simulink model "doc_fmsampletime"  (Simulink 5.0)
settings: Solver=ode45  StartTime=0.0  StopTime=10.0  RelTol=1e-3
undefined symbols (not defined in the file): slcm
libraries: commanapbnd2 x1
settings Model: CovMetricSettings=d  Creator=agaltman  LastModifiedBy=agaltman  SignalLoggingName=logsOut  BlockReductionOpt=off  BooleanDataType=off  ZeroCrossControl=UseLocalSettings  RTWMathFcnLibMatFile=iso_c_tmw.mat

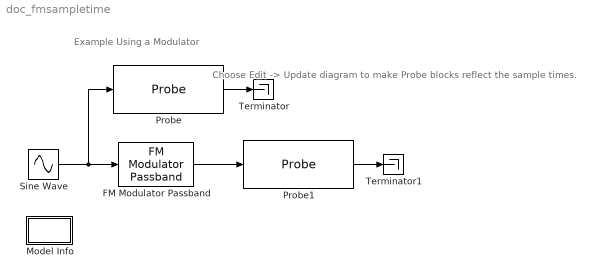
== system doc_fmsampletime ==
  note: Example Using a Modulator
  note: Choose Edit -> Update diagram
      | to make Probe blocks reflect
      | the sample times.
  FM Modulator Passband : commanapbnd2/FM Modulator Passband  Fc=100  Ph=0  HzPerV=1  ts=1  td=Inf
  Model Info : Subsystem  LoadFcn=slcm LoadBlock;  InitFcn=slcm('UpdateAllCMBlocksInThisModelInit')  mask(CMBlock){InitialSaveTempField=, InitialBlockCM=none, BlockCM=none, Frame=on, SaveTempField=, DisplayStringWithTags=Info, MaskDisplayString=Info, HorizontalTextAlignment=Center, LeftAlignmentValue=0.5, SourceBlockDiagram=doc_fmsampletime, TagMaxNumber=20, CMTag1=, CMTag2=, CMTag3=, CMTag4=, CMTag5=, CMTag6=, CMTag7=, CMTag8=, CMTag9=, CMTag10=, CMTag11=, CMTag12=, CMTag13=, CMTag14=, CMTag15=, CMTag16=, CMTag17=, CMTag18=, CMTag19=, CMTag20=}
      mask help: This block allows revision control information to be displayed within the model.
      settings: CopyFcn=slcm CopyBlock;  DeleteFcn=slcm Cancel;  PostSaveFcn=slcm('UpdateAllCMBlocksInThisModel')  NameChangeFcn=slcm Rename;  OpenFcn=commdemohelp;
      mask Display: text(str2num(LeftAlignmentValue), 0.5, MaskDisplayString, 'HorizontalAlignment', HorizontalTextAlignment)
  Probe : Probe  ProbeWidth=off  ProbeComplexSignal=off
  Probe1 : Probe  ProbeWidth=off  ProbeComplexSignal=off
  Sine Wave : Sin  SampleTime=1
  Terminator : Terminator
  Terminator1 : Terminator
  wires:
  Sine Wave/1 -> Probe/1, FM Modulator Passband/1
  FM Modulator Passband/1 -> Probe1/1
  Probe/1 -> Terminator/1
  Probe1/1 -> Terminator1/1

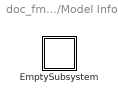
== system doc_fmsampletime/Model Info ==
  EmptySubsystem : Subsystem

== system doc_fmsampletime/Model Info/EmptySubsystem ==
